simulink model "module1model1"  (R2022b)
settings: Solver=FixedStepAuto  StartTime=0.0  StopTime=20  FixedStep=0.1  RelTol=1e-3
undefined symbols (not defined in the file): Design, Pre
settings Model: Creator=nnakhjiri  LastModifiedBy=nnakhjiri

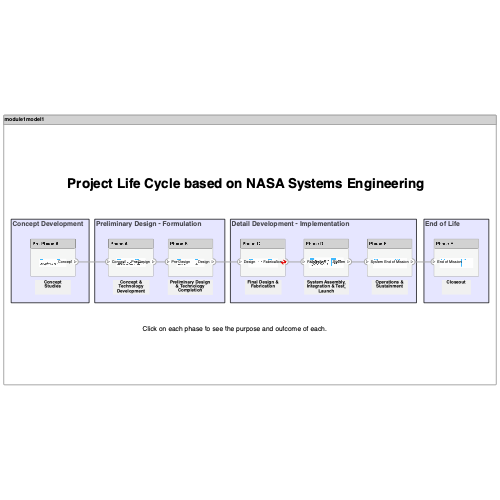
[thumbnail: Simulink's stored preview of the top-level diagram]
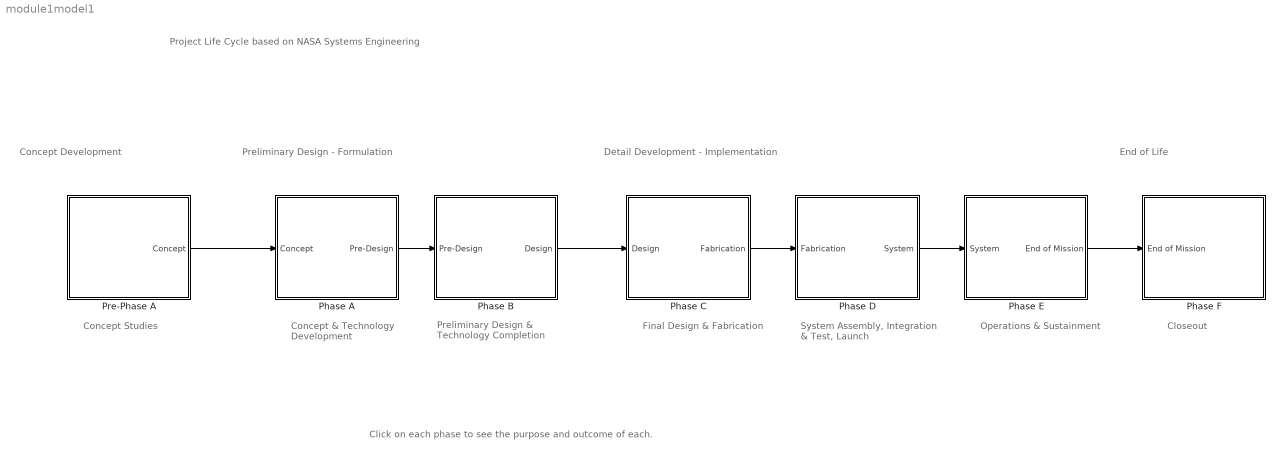
== system module1model1 ==
  note: Click on each phase to see the purpose and outcome of each.
  note: Project Life Cycle based on NASA Systems Engineering
  note: Concept Studies
  note: End of Life
  note: Detail Development - Implementation
  note: Preliminary Design - Formulation
  note: Concept Development
  note: Concept & Technology Development
  note: Preliminary Design & Technology Completion
  note: Final Design & Fabrication
  note: System Assembly, Integration & Test, Launch
  note: Operations & Sustainment
  note: Closeout
  Phase A : Subsystem
      settings: PortSchema="{\"entries\":[{\"content\":{\"headerSize\":26,\"margin\":15,\"minimumSpacing\":25,\"sides\":[{\"content\":{\"connectorIds\":[\"In1\"]},\"type\":\"ConnectorPlacement.EquallySpacedRectSide\",\"uuid\":\"109f93b1-a395-4562-8cdd-9be1fcba379d\"},{\"content\":{\"connectorIds\":[\"Out1\"],\"side\":\"RIGHT\"},\"type\":\"ConnectorPlacement.EquallySpacedRectSide\",\"uuid\":\"758d0282-9e92-4869-90e7-c9269f99ebb6\"},{\"content\":{\"connectorIds\":[],\"side\":\"TOP\"},\"type\":\"ConnectorPlacement.EquallySpacedRectSide\",\"uuid\":\"20615ce1-71a5-43a8-8714-4dc16148907e\"}]},\"type\":\"ConnectorPlacement.EquallySpacedConnector\",\"uuid\":\"0dfb5f2a-a83b-489e-875f-0b8dd509abd6\"}],\"packageUris\":[\"http://schema.mathworks.com/mf0/Connector/R2020b\"],\"version\":\"1.0\"}"
  Phase B : Subsystem
      settings: PortSchema="{\"entries\":[{\"content\":{\"headerSize\":26,\"margin\":15,\"minimumSpacing\":25,\"sides\":[{\"content\":{\"connectorIds\":[\"In1\"]},\"type\":\"ConnectorPlacement.EquallySpacedRectSide\",\"uuid\":\"109f93b1-a395-4562-8cdd-9be1fcba379d\"},{\"content\":{\"connectorIds\":[\"Out1\"],\"side\":\"RIGHT\"},\"type\":\"ConnectorPlacement.EquallySpacedRectSide\",\"uuid\":\"758d0282-9e92-4869-90e7-c9269f99ebb6\"},{\"content\":{\"connectorIds\":[],\"side\":\"TOP\"},\"type\":\"ConnectorPlacement.EquallySpacedRectSide\",\"uuid\":\"20615ce1-71a5-43a8-8714-4dc16148907e\"}]},\"type\":\"ConnectorPlacement.EquallySpacedConnector\",\"uuid\":\"0dfb5f2a-a83b-489e-875f-0b8dd509abd6\"}],\"packageUris\":[\"http://schema.mathworks.com/mf0/Connector/R2020b\"],\"version\":\"1.0\"}"
  Phase C : Subsystem
      settings: PortSchema="{\"entries\":[{\"content\":{\"headerSize\":26,\"margin\":15,\"minimumSpacing\":25,\"sides\":[{\"content\":{\"connectorIds\":[\"In1\"]},\"type\":\"ConnectorPlacement.EquallySpacedRectSide\",\"uuid\":\"109f93b1-a395-4562-8cdd-9be1fcba379d\"},{\"content\":{\"connectorIds\":[\"Out1\"],\"side\":\"RIGHT\"},\"type\":\"ConnectorPlacement.EquallySpacedRectSide\",\"uuid\":\"758d0282-9e92-4869-90e7-c9269f99ebb6\"},{\"content\":{\"connectorIds\":[],\"side\":\"TOP\"},\"type\":\"ConnectorPlacement.EquallySpacedRectSide\",\"uuid\":\"20615ce1-71a5-43a8-8714-4dc16148907e\"}]},\"type\":\"ConnectorPlacement.EquallySpacedConnector\",\"uuid\":\"0dfb5f2a-a83b-489e-875f-0b8dd509abd6\"}],\"packageUris\":[\"http://schema.mathworks.com/mf0/Connector/R2020b\"],\"version\":\"1.0\"}"
  Phase D : Subsystem
      settings: PortSchema="{\"entries\":[{\"content\":{\"headerSize\":26,\"margin\":15,\"minimumSpacing\":25,\"sides\":[{\"content\":{\"connectorIds\":[\"In1\"]},\"type\":\"ConnectorPlacement.EquallySpacedRectSide\",\"uuid\":\"109f93b1-a395-4562-8cdd-9be1fcba379d\"},{\"content\":{\"connectorIds\":[\"Out1\"],\"side\":\"RIGHT\"},\"type\":\"ConnectorPlacement.EquallySpacedRectSide\",\"uuid\":\"758d0282-9e92-4869-90e7-c9269f99ebb6\"},{\"content\":{\"connectorIds\":[],\"side\":\"TOP\"},\"type\":\"ConnectorPlacement.EquallySpacedRectSide\",\"uuid\":\"20615ce1-71a5-43a8-8714-4dc16148907e\"}]},\"type\":\"ConnectorPlacement.EquallySpacedConnector\",\"uuid\":\"0dfb5f2a-a83b-489e-875f-0b8dd509abd6\"}],\"packageUris\":[\"http://schema.mathworks.com/mf0/Connector/R2020b\"],\"version\":\"1.0\"}"
  Phase E : Subsystem
      settings: PortSchema="{\"entries\":[{\"content\":{\"headerSize\":26,\"margin\":15,\"minimumSpacing\":25,\"sides\":[{\"content\":{\"connectorIds\":[\"In1\"]},\"type\":\"ConnectorPlacement.EquallySpacedRectSide\",\"uuid\":\"109f93b1-a395-4562-8cdd-9be1fcba379d\"},{\"content\":{\"connectorIds\":[\"Out1\"],\"side\":\"RIGHT\"},\"type\":\"ConnectorPlacement.EquallySpacedRectSide\",\"uuid\":\"758d0282-9e92-4869-90e7-c9269f99ebb6\"},{\"content\":{\"connectorIds\":[],\"side\":\"TOP\"},\"type\":\"ConnectorPlacement.EquallySpacedRectSide\",\"uuid\":\"20615ce1-71a5-43a8-8714-4dc16148907e\"}]},\"type\":\"ConnectorPlacement.EquallySpacedConnector\",\"uuid\":\"0dfb5f2a-a83b-489e-875f-0b8dd509abd6\"}],\"packageUris\":[\"http://schema.mathworks.com/mf0/Connector/R2020b\"],\"version\":\"1.0\"}"
  Phase F : Subsystem
      settings: PortSchema="{\"entries\":[{\"content\":{\"headerSize\":26,\"margin\":15,\"minimumSpacing\":25,\"sides\":[{\"content\":{\"connectorIds\":[\"In1\"]},\"type\":\"ConnectorPlacement.EquallySpacedRectSide\",\"uuid\":\"109f93b1-a395-4562-8cdd-9be1fcba379d\"},{\"content\":{\"connectorIds\":[],\"side\":\"RIGHT\"},\"type\":\"ConnectorPlacement.EquallySpacedRectSide\",\"uuid\":\"758d0282-9e92-4869-90e7-c9269f99ebb6\"},{\"content\":{\"connectorIds\":[],\"side\":\"TOP\"},\"type\":\"ConnectorPlacement.EquallySpacedRectSide\",\"uuid\":\"20615ce1-71a5-43a8-8714-4dc16148907e\"},{\"content\":{\"connectorIds\":[],\"side\":\"BOTTOM\"},\"type\":\"ConnectorPlacement.EquallySpacedRectSide\",\"uuid\":\"b756fc2d-5f5f-4706-ba0e-3a4504bff326\"}]},\"type\":\"ConnectorPlacement.EquallySpacedConnector\",\"uuid\":\"0dfb5f2a-a83b-489e-875f-0b8dd509abd6\"}],\"packageUris\":[\"http://schema.mathworks.com/mf0/Connector/R2020b\"],\"version\":\"1.0\"}"
  Pre-Phase A : Subsystem
      settings: PortSchema="{\"entries\":[{\"content\":{\"headerSize\":26,\"margin\":15,\"minimumSpacing\":25,\"sides\":[{\"content\":{\"connectorIds\":[]},\"type\":\"ConnectorPlacement.EquallySpacedRectSide\",\"uuid\":\"109f93b1-a395-4562-8cdd-9be1fcba379d\"},{\"content\":{\"connectorIds\":[\"Out1\"],\"side\":\"RIGHT\"},\"type\":\"ConnectorPlacement.EquallySpacedRectSide\",\"uuid\":\"758d0282-9e92-4869-90e7-c9269f99ebb6\"},{\"content\":{\"connectorIds\":[],\"side\":\"TOP\"},\"type\":\"ConnectorPlacement.EquallySpacedRectSide\",\"uuid\":\"20615ce1-71a5-43a8-8714-4dc16148907e\"}]},\"type\":\"ConnectorPlacement.EquallySpacedConnector\",\"uuid\":\"0dfb5f2a-a83b-489e-875f-0b8dd509abd6\"}],\"packageUris\":[\"http://schema.mathworks.com/mf0/Connector/R2020b\"],\"version\":\"1.0\"}"
  wires:
  Phase A/1(Pre-Design) -> Phase B/1(Pre-Design)
  Phase D/1(System) -> Phase E/1(System)
  ? -> ?
  Phase B/1(Design) -> Phase C/1(Design)
  Pre-Phase A/1(Concept) -> Phase A/1(Concept)
  Phase E/1(End of Mission) -> Phase F/1(End of Mission)
  Phase C/1(Fabrication) -> Phase D/1(Fabrication)

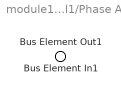
== system module1model1/Phase A ==
  Bus Element In1 : Inport  PortName=Concept
  Bus Element Out1 : Outport  PortName=Pre-Design

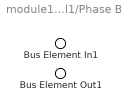
== system module1model1/Phase B ==
  Bus Element In1 : Inport  PortName=Pre-Design
  Bus Element Out1 : Outport  PortName=Design

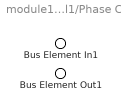
== system module1model1/Phase C ==
  Bus Element In1 : Inport  PortName=Design
  Bus Element Out1 : Outport  PortName=Fabrication

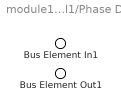
== system module1model1/Phase D ==
  Bus Element In1 : Inport  PortName=Fabrication
  Bus Element Out1 : Outport  PortName=System

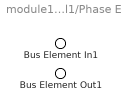
== system module1model1/Phase E ==
  Bus Element In1 : Inport  PortName=System
  Bus Element Out1 : Outport  PortName=End of Mission

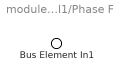
== system module1model1/Phase F ==
  Bus Element In1 : Inport  PortName=End of Mission

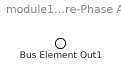
== system module1model1/Pre-Phase A ==
  Bus Element Out1 : Outport  PortName=Concept
